simulink model "CaseNode2"  (R2023b)
settings: Solver=VariableStepAuto  StartTime=0.0  StopTime=10.0  RelTol=1e-3
settings Model: Creator=jsonm  LastModifiedBy=jsonm

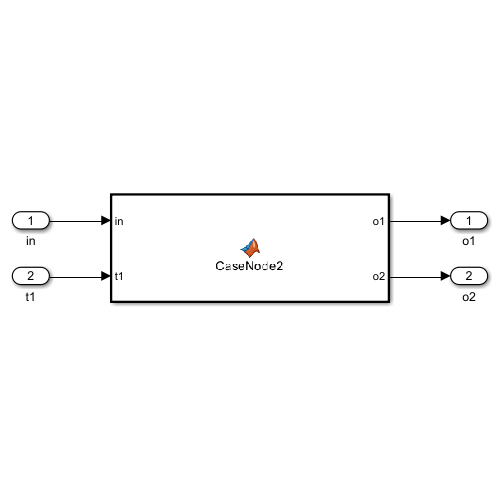
[thumbnail: Simulink's stored preview of the top-level diagram]
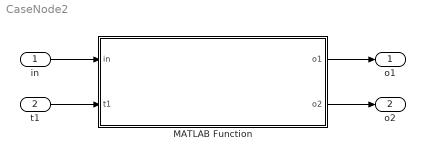
== system CaseNode2 ==
  in : Inport
  t1 : Inport  Port=2
  MATLAB Function : MATLAB Function  TreatAsAtomicUnit=on
  o1 : Outport
  o2 : Outport  Port=2
  wires:
  MATLAB Function/1(o1) -> o1/1
  MATLAB Function/2(o2) -> o2/1
  in/1 -> MATLAB Function/1(in)
  t1/1 -> MATLAB Function/2(t1)

== matlab function CaseNode2/MATLAB Function ==
  data: in input; o1 output; t1 input; o2 output
function [o1, o2] = CaseNode2(in, t1)

% Method to demux input into one of 2 possible outputs based on
% probabilities
%
% t1 is a threshold bound between 0 and 100 used as follows
% x = rand*100
% 0 <= x < t1 => o1
%
% Negative is a non-valid output
%
% Written by Darian Muresan

o1 = -1;
o2 = -1;

% generate a random signal with magnitude 100x = random*100;
x = rand*100;
if (0 <= x && x <= t1)
    o1 = in;
else
    o2 = in;
end
